simulink model "usrp_tx"  (R2014b)
settings: Solver=ode45  StartTime=0.0  StopTime=inf  RelTol=1e-3
libraries: siglabs_lib x1, commrandsrc2 x1, commsdrhw_v2 x1
settings Model: Creator=Ben  LastModifiedBy=Ben

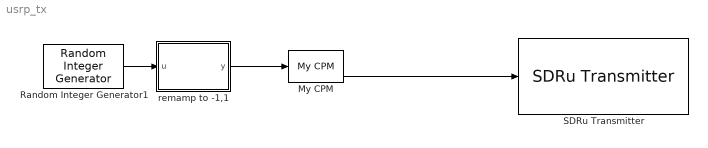
== system usrp_tx ==
  My CPM : siglabs_lib/My CPM  SampsPerSym=10  RotationsPerSym=1  FilterBufferLength=3  ClockUpDownFrequency=100
  Random Integer Generator1 : commrandsrc2/Random Integer Generator  mul=2  seed=42  Ts=5.1200e-05  frameBased=off  sampPerFrame=1024  orient=off  outDataType=double
  SDRu Transmitter : commsdrhw_v2/SDRu Transmitter  rxtx=tx  platform=N200/N210/USRP2  USRP2_IP='192.168.10.2'  USRP_IP_X300='192.168.10.2'  USRP_IP_X310='192.168.10.2'  USRP_serialNumB200=''  USRP_serialNumB210=''  centerFrequency=915E6  centerFrequencySrc=Dialog  loOffset=0  loOffsetSrc=Dialog  masterClkRateB200=32e6  masterClkRateB210=32e6  masterClkRateX300=200e6  masterClkRateX310=200e6  masterClkRateParam=100e6  gain=8  gainSrc=Dialog  decimInterp=512  decimInterpSrc=Dialog  USRP2_IP_NUM=[49 57 50 46 49 54 56 46 49 48 46 50]  frameLength=362  outputDatatype=int16  overrunUnderrunPort=off  sampleTime=1  dboardInfo=|  HOST_DATA_PORT=30000  HOST_CONTROL_PORT=30001  USRP2_DATA_PORT=32769  USRP2_CONTROL_PORT=32768  bufferMode=Guaranteed contiguous buffer  EnableBurstMode=on  NumFramesInBurst=40000  USRP_ID='192.168.10.2'
      | dbid: 0
      |           dbName: 'no db found'
      |          freqMin: 0
      |          freqMax: 0
      |          gainMin: 0
      |          gainMax: 0
      |     gainStepSize: 0
  remamp to -1,1 : MATLAB Function  TreatAsAtomicUnit=on
  wires:
  Random Integer Generator1/1 -> remamp to -1,1/1(u)
  remamp to -1,1/1(y) -> My CPM/1
  My CPM/3 -> SDRu Transmitter/1

== matlab function usrp_tx/remamp to -1,1 ==
  data: u input; y output
function y = fcn(u)
%#codegen

y = (u*2)-1;
